simulink model "untitled"  (R2020b)
settings: Solver=VariableStepAuto  StartTime=0.0  StopTime=200  RelTol=1e-2
values from neighbouring files (symbols this model uses):
  I_inv = inv(I)    [SixDOFModel.m]    (also in initializeParameters.m; nonlinear_model6DOF.m = globalParameters.I_inv)
  m = 9300    [OnePointOfMassModel.m]    (also in SixDOFModel.m = 120000; coupling_control.m = i-1; defineABC.m = size(B_1,2) + size(B_2,2); implicit_linmod.m = length(U_ap))
  Omega_init = [0;0;0]    [SixDOFModel.m]
  P_e_init = [0;0;1000]    [SixDOFModel.m]
  Phi_init = [pi/20;0;pi/10]    [SixDOFModel.m]
  V_init = [100;0;10]    [SixDOFModel.m]
settings Model: Creator=teteu  LastModifiedBy=teteu

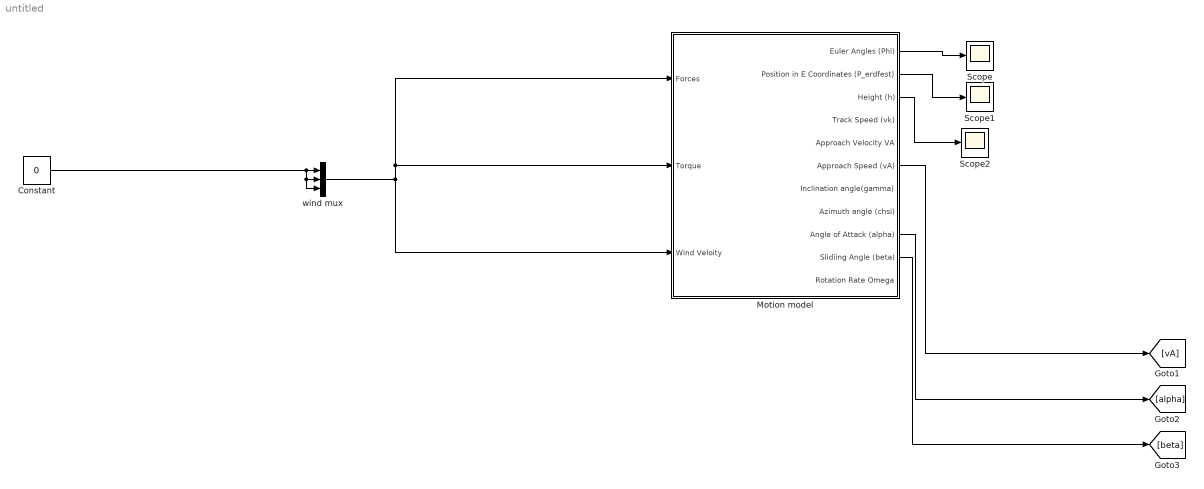
== system untitled ==
  Constant : Constant  Value=0
  "Motion model " : Subsystem
  Scope : Scope
  Scope1 : Scope
  Scope2 : Scope
  wind mux : Mux  Inputs=3
  wires:
  Constant/1 -> wind mux/3, wind mux/2, wind mux/1
  "Motion model "/10(Slidiing Angle (beta)) -> [beta]
  "Motion model "/6(Approach Speed (vA)) -> [vA]
  "Motion model "/1(Euler Angles (Phi)) -> Scope/1
  wind mux/1 -> "Motion model "/2(Torque), "Motion model "/1(Forces), "Motion model "/3(Wind Veloity)
  "Motion model "/9(Angle of Attack (alpha)) -> [alpha]
  "Motion model "/2(Position in E Coordinates (P_erdfest)) -> Scope1/1
  "Motion model "/3(Height (h)) -> Scope2/1

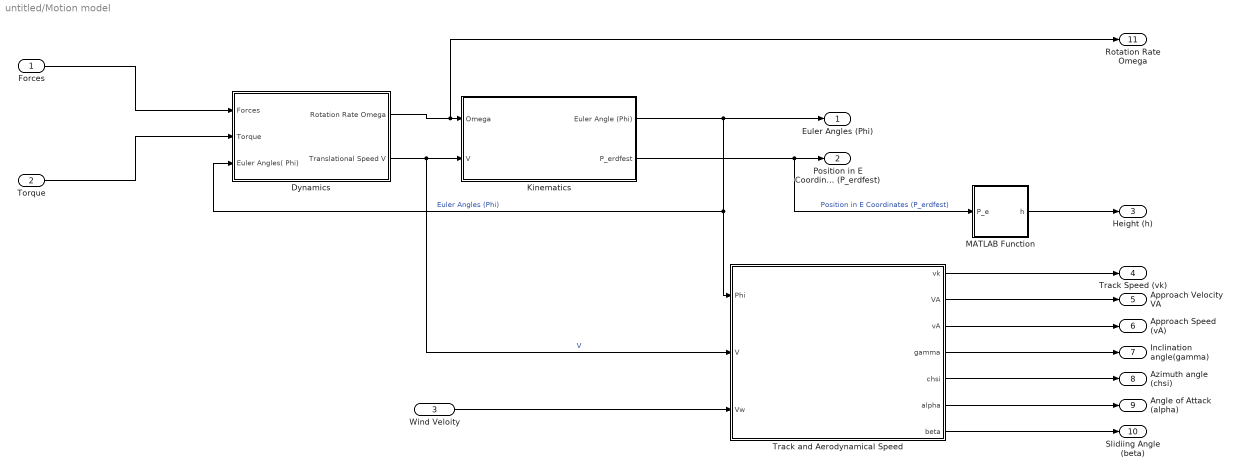
== system untitled/Motion model  ==
  Forces : Inport
  Torque : Inport  Port=2
  Wind Veloity : Inport  Port=3
  Dynamics : Subsystem
  Kinematics : Subsystem
  MATLAB Function : MATLAB Function  TreatAsAtomicUnit=on
  Track and Aerodynamical Speed : MATLAB Function  TreatAsAtomicUnit=on
  Euler Angles (Phi) : Outport
  Position in E Coordinates (P_erdfest) : Outport  Port=2
  Height (h) : Outport  Port=3
  Track Speed (vk) : Outport  Port=4
  Approach Velocity VA : Outport  Port=5
  Approach Speed (vA) : Outport  Port=6
  Inclination angle(gamma) : Outport  Port=7
  Azimuth angle (chsi) : Outport  Port=8
  Angle of Attack (alpha) : Outport  Port=9
  Slidiing Angle (beta) : Outport  Port=10
  Rotation Rate Omega : Outport  Port=11
  wires:
  Torque/1 -> Dynamics/2(Torque)
  Kinematics/1(Euler Angle (Phi)) -> Euler Angles (Phi)/1, Track and Aerodynamical Speed/1(Phi), Dynamics/3(Euler Angles( Phi))  "Euler Angles (Phi)"
  Kinematics/2(P_erdfest) -> MATLAB Function/1(P_e), Position in E Coordinates (P_erdfest)/1  "Position in E Coordinates (P_erdfest)"
  Dynamics/2(Translational Speed V) -> Track and Aerodynamical Speed/2(V), Kinematics/2(V)  "V"
  Forces/1 -> Dynamics/1(Forces)
  Dynamics/1(Rotation Rate Omega) -> Rotation Rate Omega/1, Kinematics/1(Omega)
  Track and Aerodynamical Speed/1(vk) -> Track Speed (vk)/1
  Track and Aerodynamical Speed/3(vA) -> Approach Speed (vA)/1
  Track and Aerodynamical Speed/4(gamma) -> Inclination angle(gamma)/1
  Track and Aerodynamical Speed/5(chsi) -> Azimuth angle (chsi)/1
  Track and Aerodynamical Speed/6(alpha) -> Angle of Attack (alpha)/1
  Track and Aerodynamical Speed/7(beta) -> Slidiing Angle (beta)/1
  Wind Veloity/1 -> Track and Aerodynamical Speed/3(Vw)
  MATLAB Function/1(h) -> Height (h)/1
  Track and Aerodynamical Speed/2(VA) -> Approach Velocity VA/1

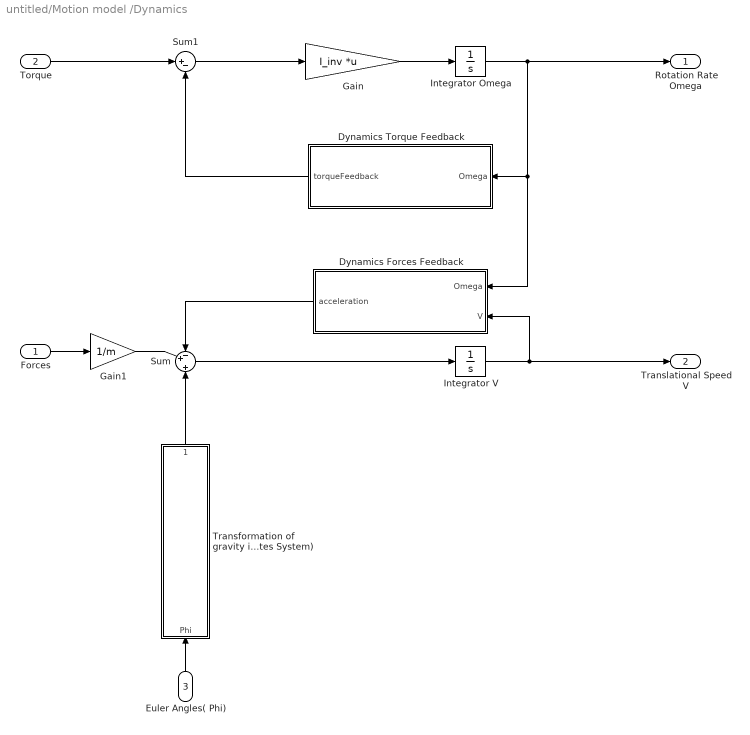
== system untitled/Motion model /Dynamics ==
  Forces : Inport
  Torque : Inport  Port=2
  Euler Angles( Phi) : Inport  Port=3
  Dynamics Forces Feedback : MATLAB Function  TreatAsAtomicUnit=on
  Dynamics Torque Feedback : MATLAB Function  TreatAsAtomicUnit=on
  Gain : Gain  Gain=I_inv  Multiplication=Matrix(K*u) (u vector)
  Gain1 : Gain  Gain=1/m
  Integrator Omega : Integrator  InitialCondition=Omega_init
  Integrator V : Integrator  InitialCondition=V_init
  Sum : Sum  Inputs=-+|+
  Sum1 : Sum  Inputs=|+-
  Transformation of gravity in (Körperfestes System) : MATLAB Function  TreatAsAtomicUnit=on
  Rotation Rate Omega : Outport
  Translational Speed V : Outport  Port=2
  wires:
  Euler Angles( Phi)/1 -> Transformation of gravity in (Körperfestes System)/1(Phi)
  Transformation of gravity in (Körperfestes System)/1(gravityAcceleration) -> Sum/3
  Forces/1 -> Gain1/1
  Sum/1 -> Integrator V/1
  Integrator V/1 -> Translational Speed V/1, Dynamics Forces Feedback/2(V)
  Gain1/1 -> Sum/2
  Dynamics Forces Feedback/1(acceleration) -> Sum/1
  Torque/1 -> Sum1/1
  Sum1/1 -> Gain/1
  Gain/1 -> Integrator Omega/1
  Integrator Omega/1 -> Dynamics Forces Feedback/1(Omega), Dynamics Torque Feedback/1(Omega), Rotation Rate Omega/1
  Dynamics Torque Feedback/1(torqueFeedback) -> Sum1/2

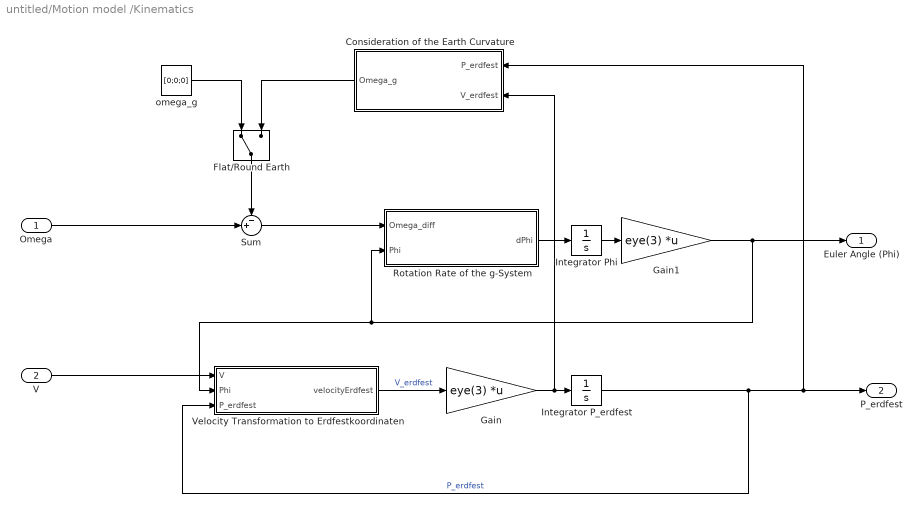
== system untitled/Motion model /Kinematics ==
  Omega : Inport
  V : Inport  Port=2
  Consideration of the Earth Curvature : MATLAB Function  TreatAsAtomicUnit=on
  Flat/Round Earth : ManualSwitch
  Gain : Gain  Gain=eye(3)  Multiplication=Matrix(K*u) (u vector)
  Gain1 : Gain  Gain=eye(3)  Multiplication=Matrix(K*u) (u vector)
  Integrator P_erdfest : Integrator  InitialCondition=P_e_init
  Integrator Phi : Integrator  InitialCondition=Phi_init
  Rotation Rate of the g-System : MATLAB Function  TreatAsAtomicUnit=on
  Sum : Sum  Inputs=-+|
  Velocity Transformation to Erdfestkoordinaten : MATLAB Function  TreatAsAtomicUnit=on
  omega_g : Constant  Value=[0;0;0]
  Euler Angle (Phi) : Outport
  P_erdfest : Outport  Port=2
  wires:
  Integrator P_erdfest/1 -> Consideration of the Earth Curvature/1(P_erdfest), P_erdfest/1, Velocity Transformation to Erdfestkoordinaten/3(P_erdfest)  "P_erdfest"
  Velocity Transformation to Erdfestkoordinaten/1(velocityErdfest) -> Gain/1  "V_erdfest"
  V/1 -> Velocity Transformation to Erdfestkoordinaten/1(V)
  Rotation Rate of the g-System/1(dPhi) -> Integrator Phi/1
  Gain/1 -> Consideration of the Earth Curvature/2(V_erdfest), Integrator P_erdfest/1
  Sum/1 -> Rotation Rate of the g-System/1(Omega_diff)
  Omega/1 -> Sum/2
  Integrator Phi/1 -> Gain1/1
  Gain1/1 -> Rotation Rate of the g-System/2(Phi), Velocity Transformation to Erdfestkoordinaten/2(Phi), Euler Angle (Phi)/1
  omega_g/1 -> Flat/Round Earth/1
  Flat/Round Earth/1 -> Sum/1
  Consideration of the Earth Curvature/1(Omega_g) -> Flat/Round Earth/2

== matlab function untitled/Motion model /Dynamics/Dynamics Forces Feedback ==
  data: Omega input; V input; acceleration output; Omega_e_tilde parameter
function acceleration = accelerationFeedback(Omega,V,Omega_e_tilde)
Omega_tilde = vecToMat(Omega);
acceleration = (Omega_tilde + Omega_e_tilde)*V;

== matlab function untitled/Motion model /Dynamics/Transformation of gravity in (Körperfestes System) ==
  data: Phi input; gravityAcceleration output; g parameter
function gravityAcceleration = Tfg(Phi,g)
G = [0;0;g]; %Graviation vector in geodetic ref. Frame
Tfg = coordTransfMatrix(Phi(1),1)*coordTransfMatrix(Phi(2),2)*coordTransfMatrix(Phi(3),3); % Transformation Matrix goedetic --> body reference Frame
gravityAcceleration = Tfg*G;

== matlab function untitled/Motion model /Dynamics/Dynamics Torque Feedback ==
  data: Omega input; torqueFeedback output; I parameter
function torqueFeedback = getTorqueFeedback(Omega,I)
Omega_tilde = vecToMat(Omega);
help = Omega_tilde*I;
torqueFeedback = help*Omega;

== matlab function untitled/Motion model /Kinematics/Velocity Transformation to Erdfestkoordinaten ==
  data: V input; Phi input; velocityErdfest output; P_erdfest input
function velocityErdfest = Tef(V,Phi,P_erdfest)
%Converts the velocity from Körper to Erdfest Koordinaten
%Phi: Vector w. Euler Angles
% P_erdfest: Position Vector 
lambda = atan2(P_erdfest(2),P_erdfest(1)); %Angle Längengrad
sigma = asin(P_erdfest(3)/sqrt(P_erdfest(1)^2+P_erdfest(2)^2+P_erdfest(3)^2)); %Declination Angle 
TgE = coordTransfMatrix(-pi/2 - sigma,2)*coordTransfMatrix(lambda,3);
Tfg = coordTransfMatrix(Phi(1),1)*coordTransfMatrix(Phi(2),2)*coordTransfMatrix(Phi(3),3); % Transformation Matrix goedetic --> body reference Frame
TfE = Tfg*TgE;
TEf= TfE';
velocityErdfest = TEf*V;

== matlab function untitled/Motion model /Kinematics/Rotation Rate of the g-System ==
  data: Omega_diff input; dPhi output; Phi input
function dPhi = J(Omega_diff,Phi)
%Rotation rate of the g-system depending on the euler angles
%Phi: euler Angles
%Omega_ diff = Omega-Omega_g
%dPhi: Rotaion Speed considering the rotation rate of the geodathic system
phi = Phi(1);
theta = Phi(2);
J = 1/cos(theta)*[cos(theta) sin(phi)*sin(theta) cos(phi)*sin(theta) ;0 cos(phi)*cos(theta) -sin(phi)*cos(theta);0 sin(phi) cos(phi)];
dPhi = J*Omega_diff;

== matlab function untitled/Motion model /Kinematics/Consideration of the Earth Curvature ==
  data: P_erdfest input; V_erdfest input; Omega_g output; omega_e parameter
function Omega_g = fcn(P_erdfest, V_erdfest, omega_e)
%Calculation of the rotation speed of the geodatic system caused by the
%curve of the earth. Omega_g = 0 for flat earth.
lambda = atan2(P_erdfest(2),P_erdfest(1)); %Angle Längengrad
sigma = asin(P_erdfest(3)/sqrt(P_erdfest(1)^2+P_erdfest(2)^2+P_erdfest(3)^2)); %Declination Angle


TgE = coordTransfMatrix(pi/2 - sigma,2)*coordTransfMatrix(lambda,3);
V_geod = TgE*V_erdfest;
P_geod = TgE*P_erdfest;
r = P_geod(3); % Warning !!! r IS GIERRATE AND NOT A POSITION
dsigma = V_geod(1)/r;
dlambda = V_geod(2)/(cos(sigma)*r);

Omega_g = [cos(sigma);0;-sin(sigma)]*(omega_e+ dlambda)+[0;-dsigma;0];

== matlab function untitled/Motion model /Track and Aerodynamical Speed ==
  data: Phi input; V input; vk output; VA output; vA output; gamma output; chsi output; alpha output; beta output; Vw input
function [vk,VA,vA, gamma, chsi,alpha,beta] = getTrackAndAero(Phi,V,Vw)
%Get The Track Speed, the Approach Speed, the inclinational angle ,
%the Azimuth angle, the angle of attack and the Sliding angle from the
%Speed from the Translational Velocity. 
Tfg = coordTransfMatrix(Phi(1),1)*coordTransfMatrix(Phi(2),2)*coordTransfMatrix(Phi(3),3); % Transformation Matrix goedetic --> body reference Frame
Tgf = Tfg';
Vk = Tgf*V; %Track Velocity
vk = sqrt(Vk(1)^2+Vk(2)^2+Vk(3)^2); %Track Speed [m/s]
gamma = -asin(Vk(3)/vk); %Inclination Angle [rad]
chsi = atan2(Vk(2),Vk(1));
VA = V - Tfg*Vw; %Approach Speed
vA = sqrt(VA(1)^2+VA(2)^2+VA(3)^2); %Approach Speed [m/s]
alpha = atan(VA(3)/VA(1)); % Angle of attck [m/s]
beta = asin(VA(2)/vA);

== matlab function untitled/Motion model /MATLAB Function ==
  data: P_e input; h output
function h = getHeight(P_e)
h = P_e(3);
